simulink model "etc_demo_simc"  (R2017a)
settings: Solver=VariableStepAuto  StartTime=0.0  StopTime=3  RelTol=1e-3
values from neighbouring files (symbols this model uses):
  B = 0.0088    [sim_demo_set_para.m]
  J = 0.0021    [sim_demo_set_para.m]
  K = 0.383    [sim_demo_set_para.m]
  Ks = 0.087    [sim_demo_set_para.m]
  L = 1.5e-3    (= 0.0015)    [sim_demo_set_para.m]
  R = 1.5    [sim_demo_set_para.m]
  Tpl = 0.396    [sim_demo_set_para.m]
libraries: fl_lib x12, nesl_utility x5, simulink x1
settings Model: Creator=xiaopan-local  LastModifiedBy=xiaopan

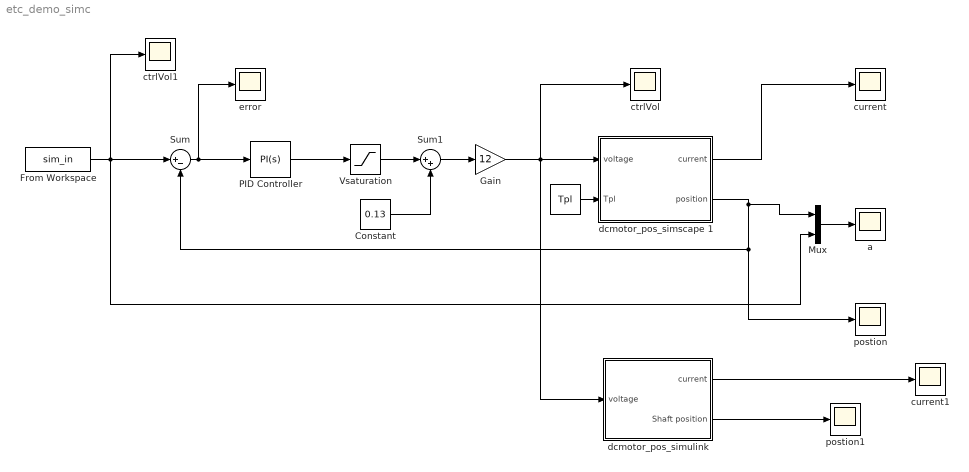
== system etc_demo_simc ==
  " " : Constant  Value=Tpl
  Constant : Constant  Value=0.13
  From Workspace : FromWorkspace  VariableName=sim_in  OutDataTypeStr=double  SampleTime=0  OutputAfterFinalValue=Holding final value
  Gain : Gain  Gain=12
  Mux : Mux  Inputs=2
  PID Controller : simulink/Continuous/PID Controller  Controller=PI  TimeDomain=Continuous-time  SampleTime=-1  IntegratorMethod=Forward Euler  FilterMethod=Forward Euler  Form=Parallel  UseFilter=on  ControllerParametersSource=internal  P=0.8  I=0.4  D=0.1  N=1000  InitialConditionSource=internal  InitialConditionForIntegrator=0  InitialConditionForFilter=0  ExternalReset=none  LimitOutput=off  UpperSaturationLimit=1  LowerSaturationLimit=0  LinearizeAsGain=on  AntiWindupMode=none  Kb=1  TrackingMode=off  Kt=1  PParamMin=[]  PParamMax=[]  IParamMin=[]  IParamMax=[]  DParamMin=[]  DParamMax=[]  NParamMin=[]  NParamMax=[]  KbParamMin=[]  KbParamMax=[]  KtParamMin=[]  KtParamMax=[]  POutMin=[]  POutMax=[]  IOutMin=[]  IOutMax=[]  DOutMin=[]  DOutMax=[]  NOutMin=[]  NOutMax=[]  KbOutMin=[]  KbOutMax=[]  KtOutMin=[]  KtOutMax=[]  IntegratorOutMin=[]  IntegratorOutMax=[]  FilterOutMin=[]  FilterOutMax=[]  SumOutMin=[]  SumOutMax=[]  SumI1OutMin=[]  SumI1OutMax=[]  SumI2OutMin=[]  SumI2OutMax=[]  SumI3OutMin=[]  SumI3OutMax=[]  SumDOutMin=[]  SumDOutMax=[]  SaturationOutMin=[]  SaturationOutMax=[]  IntegratorContinuousStateAttributes=''  IntegratorStateMustResolveToSignalObject=off  IntegratorRTWStateStorageClass=Auto  FilterContinuousStateAttributes=''  FilterStateMustResolveToSignalObject=off  FilterRTWStateStorageClass=Auto  DifferentiatorICPrevScaledInput=0  DifferentiatorOutMin=[]  DifferentiatorOutMax=[]  InitialConditionSetting=State (most efficient)
  Sum : Sum  Inputs=|+-
  Sum1 : Sum  Inputs=|++
  Vsaturation : Saturate  UpperLimit=1  LowerLimit=-1
  a : Scope
  ctrlVol : Scope
  ctrlVol1 : Scope
  current : Scope
  current1 : Scope
  dcmotor_pos_simscape 1 : Subsystem
  dcmotor_pos_simulink : Subsystem
  "error " : Scope
  postion : Scope
  postion1 : Scope
  wires:
  From Workspace/1 -> ctrlVol1/1, Mux/2, Sum/1
  dcmotor_pos_simscape 1/1(current) -> current/1
  dcmotor_pos_simscape 1/2(position) -> Sum/2, postion/1, Mux/1
  " "/1 -> dcmotor_pos_simscape 1/2(Tpl)
  Mux/1 -> a/1
  Sum/1 -> "error "/1, PID Controller/1
  dcmotor_pos_simulink/2(Shaft position) -> postion1/1
  dcmotor_pos_simulink/1(current) -> current1/1
  Gain/1 -> dcmotor_pos_simulink/1(voltage), dcmotor_pos_simscape 1/1(voltage), ctrlVol/1
  PID Controller/1 -> Vsaturation/1
  Vsaturation/1 -> Sum1/1
  Sum1/1 -> Gain/1
  Constant/1 -> Sum1/2

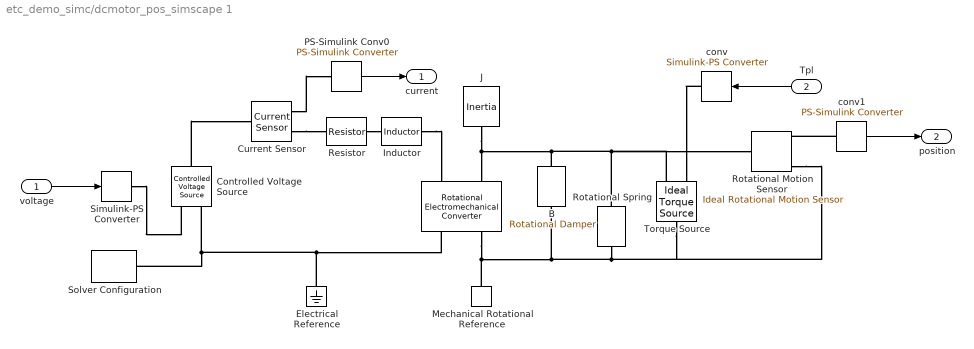
== system etc_demo_simc/dcmotor_pos_simscape 1 ==
  voltage : Inport
  Tpl : Inport  Port=2
  " " : fl_lib/Electrical/Electrical Elements/Rotational Electromechanical Converter  K=K V/(rad/s)  i_specify=off  i_priority=None  i=0 A  i_nominal_specify=off  i_nominal_unit=A  i_nominal_value=1  v_specify=off  v_priority=None  v=0 V  v_nominal_specify=off  v_nominal_unit=V  v_nominal_value=1  t_specify=off  t_priority=None  t=0 N*m  t_nominal_specify=off  t_nominal_unit=N*m  t_nominal_value=1  w_specify=off  w_priority=None  w=0 rad/s  w_nominal_specify=off  w_nominal_unit=rad/s  w_nominal_value=1
      settings: SourceProductName=Simscape
  " Rotational Motion Sensor" : fl_lib/Mechanical/Mechanical Sensors/Ideal Rotational Motion Sensor  offset=0 rad
  " Torque Source" : fl_lib/Mechanical/Mechanical Sources/Ideal Torque Source
  B : fl_lib/Mechanical/Rotational Elements/Rotational Damper  D=B N*m/(rad/s)  w_specify=off  w_priority=None  w=0 rad/s  w_nominal_specify=off  w_nominal_unit=rad/s  w_nominal_value=1  t_specify=off  t_priority=None  t=0 N*m  t_nominal_specify=off  t_nominal_unit=N*m  t_nominal_value=1
  Controlled Voltage Source : fl_lib/Electrical/Electrical Sources/Controlled Voltage Source
  Current Sensor : fl_lib/Electrical/Electrical Sensors/Current Sensor
  Electrical Reference : fl_lib/Electrical/Electrical Elements/Electrical Reference
  Inductor : fl_lib/Electrical/Electrical Elements/Inductor  l=L mH  r=0 Ohm  g=0 1/Ohm  i_specify=off  i_priority=None  i=0 A  i_nominal_specify=off  i_nominal_unit=A  i_nominal_value=1  v_specify=off  v_priority=None  v=0 V  v_nominal_specify=off  v_nominal_unit=V  v_nominal_value=1  i_L_specify=off  i_L_priority=High  i_L=0 A  i_L_nominal_specify=off  i_L_nominal_unit=A  i_L_nominal_value=1
  J : fl_lib/Mechanical/Rotational Elements/Inertia  inertia=J kg*m^2  w_specify=off  w_priority=High  w=0 rad/s  w_nominal_specify=off  w_nominal_unit=rad/s  w_nominal_value=1  t_specify=off  t_priority=None  t=0 N*m  t_nominal_specify=off  t_nominal_unit=N*m  t_nominal_value=1
      settings: LogSimulationData=on
  Mechanical Rotational Reference : fl_lib/Mechanical/Rotational Elements/Mechanical Rotational Reference
  PS-Simulink Conv0 : nesl_utility/PS-Simulink Converter  PhysicalDomain=network_engine_domain  SubClassName=ps_output  LeftPortType=input  RightPortType=output  PseudoPeriodic=off  Frequencies=[]  Unit=1  AffineConversion=off
  Resistor : fl_lib/Electrical/Electrical Elements/Resistor  R=R Ohm  i_specify=off  i_priority=None  i=0 A  i_nominal_specify=off  i_nominal_unit=A  i_nominal_value=1  v_specify=off  v_priority=None  v=0 V  v_nominal_specify=off  v_nominal_unit=V  v_nominal_value=1
  Rotational Spring : fl_lib/Mechanical/Rotational Elements/Rotational Spring  spr_rate=Ks N*m/rad  w_specify=off  w_priority=None  w=0 rad/s  w_nominal_specify=off  w_nominal_unit=rad/s  w_nominal_value=1  t_specify=off  t_priority=None  t=0 N*m  t_nominal_specify=off  t_nominal_unit=N*m  t_nominal_value=1  phi_specify=off  phi_priority=High  phi=0 rad  phi_nominal_specify=off  phi_nominal_unit=rad  phi_nominal_value=1
      settings: SourceProductName=Simscape
  Simulink-PS Converter : nesl_utility/Simulink-PS Converter  PhysicalDomain=network_engine_domain  SubClassName=ps_input  LeftPortType=input  RightPortType=output  PseudoPeriodic=off  Frequencies=[]  NoiseDistribution=none  NoiseParameters=[]  Unit=1  AffineConversion=off  FilteringAndDerivatives=provide  SimscapeFilterOrder=1  InputFilterTimeConstant=0.001  UdotUserProvided=0
  Solver Configuration : nesl_utility/Solver Configuration  PhysicalDomain=network_engine_domain  SubClassName=solver  LeftPortType=input  RightPortType=generic  Accelerate=off  Tones=[]  Harmonics=[]  SimulateNoise=off  Profile=off  UseLocalSampling=off  EnableSwitchedLinearOptims=on  FrequencyDomain=off  UseCCode=off  RelTol=0.001  AbsTol=1e-06  MinStep=1e-09  ToWorkspace=off  RevertToSquareIcSolve=off  NumHomotopyIterations=100  PhasorMode=off  PhasorModeNumHarmonics=1  OverrideAbsTol=off  DoDC=off  ResidualTolerance=1e-09  UseLocalSolver=off  LocalSolverChoice=NE_BACKWARD_EULER_ADVANCER  LocalSolverSampleTime=0.001  DoFixedCost=off  MaxNonlinIter=3  MaxModeIter=2  LinearAlgebra=Sparse  DelaysMemoryBudget=1024  AutomaticFiltering=on  FilteringTimeConstant=0.001
  conv : nesl_utility/Simulink-PS Converter  PhysicalDomain=network_engine_domain  SubClassName=ps_input  LeftPortType=input  RightPortType=output  PseudoPeriodic=off  Frequencies=[]  NoiseDistribution=none  NoiseParameters=[]  Unit=1  AffineConversion=off  FilteringAndDerivatives=provide  SimscapeFilterOrder=1  InputFilterTimeConstant=0.001  UdotUserProvided=0
  conv1 : nesl_utility/PS-Simulink Converter  PhysicalDomain=network_engine_domain  SubClassName=ps_output  LeftPortType=input  RightPortType=output  PseudoPeriodic=off  Frequencies=[]  Unit=1  AffineConversion=off
  current : Outport
  position : Outport  Port=2
  wires:
  conv1/1 -> position/1
  voltage/1 -> Simulink-PS Converter/1
  PS-Simulink Conv0/1 -> current/1
  Tpl/1 -> conv/1
  connections:
  Resistor/RConn1 -- Inductor/LConn1
  Inductor/RConn1 -- " "/LConn1
  " "/RConn2 -- " Rotational Motion Sensor"/RConn1 -- " Torque Source"/LConn1 -- Rotational Spring/LConn1 -- B/RConn1 -- Mechanical Rotational Reference/LConn1
  Electrical Reference/LConn1 -- " "/RConn1 -- Solver Configuration/RConn1 -- Controlled Voltage Source/RConn2
  conv1/LConn1 -- " Rotational Motion Sensor"/RConn3
  Current Sensor/RConn2 -- Resistor/LConn1
  Current Sensor/RConn1 -- PS-Simulink Conv0/LConn1
  Controlled Voltage Source/LConn1 -- Current Sensor/LConn1
  Simulink-PS Converter/RConn1 -- Controlled Voltage Source/RConn1
  conv/RConn1 -- " Torque Source"/RConn1
  J/LConn1 -- " Torque Source"/RConn2 -- " Rotational Motion Sensor"/LConn1 -- Rotational Spring/RConn1 -- B/LConn1 -- " "/LConn2

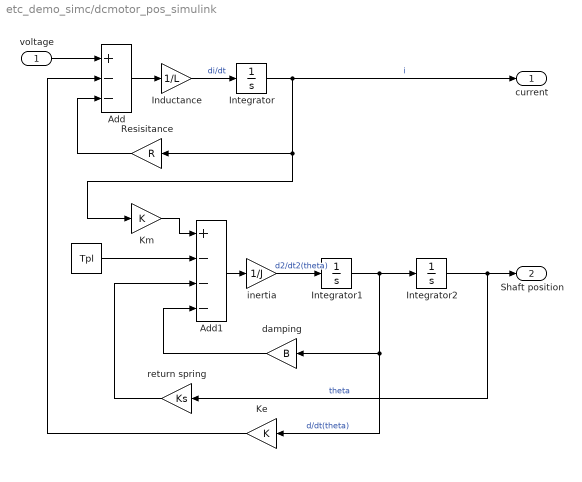
== system etc_demo_simc/dcmotor_pos_simulink ==
  voltage : Inport
  " " : Constant  Value=Tpl
  Add : Sum  Inputs=+--
  Add1 : Sum  Inputs=+---
  "Inductance " : Gain  Gain=1/L
  Integrator : Integrator
  Integrator1 : Integrator
  Integrator2 : Integrator
  Ke : Gain  Gain=K
  Km : Gain  Gain=K
  Resisitance : Gain  Gain=R
  damping : Gain  Gain=B
  inertia : Gain  Gain=1/J
  return spring : Gain  Gain=Ks
  current : Outport
  Shaft position : Outport  Port=2
  wires:
  Km/1 -> Add1/1
  Add/1 -> "Inductance "/1
  "Inductance "/1 -> Integrator/1  "di/dt"
  Integrator2/1 -> Shaft position/1, return spring/1  "theta"
  inertia/1 -> Integrator1/1  "d2/dt2(theta)"
  Integrator1/1 -> Integrator2/1, Ke/1, damping/1  "d/dt(theta)"
  Integrator/1 -> Km/1, Resisitance/1, current/1  "i"
  Add1/1 -> inertia/1
  " "/1 -> Add1/2
  Ke/1 -> Add/2
  voltage/1 -> Add/1
  Resisitance/1 -> Add/3
  return spring/1 -> Add1/3
  damping/1 -> Add1/4
